simulink model "Collision_two_cars_cs"  (Simulink 8.7)
settings: Solver=ode5  SolverMode=SingleTasking  StartTime=0.0  StopTime=inf  FixedStep=1/20  RelTol=1e-3
PreLoadFcn:
  | check_NUTS_defined;
  | 
  | assignin('base',['model_closed_' bdroot],false);
InitFcn:
  | PreScanExperimentInitFcn(bdroot)
StopFcn:
  | PreScanExperimentStopFcn(bdroot)
undefined symbols (not defined in the file): spare_1, spare_10, spare_11, spare_12, spare_13, spare_14, spare_15, spare_16, spare_17, spare_18, spare_19, spare_2, spare_3, spare_4, spare_5, spare_6, spare_7, spare_8, spare_9
libraries: PreScanSimulinkLibrary x16, PreScanUsefulBlocks x6, simulink x1
(part 2 of 3)

== system Collision_two_cars_cs/STATE_Toyota_Yaris_1 ==
  State : Inport  SampleTime=TimeStep
  Acceleration : Subsystem  mask(ToSensorWorld){PortName=Acceleration_Toyota_Yaris_1, PortIndex=60, PortWidth=3, TimeStep=1/20}
      mask prompts: PortName "Port Name [-]"; PortIndex "Index [-]"; PortWidth "Port Dimensions [-]"; TimeStep "Upload Period [s]"
      mask help: Sends signal(s) from Simulink to the Sensor World
      mask Help:
      | Sends signal(s) from Simulink to the Sensor World.
      | 
      | - Port Name [-]: specifies the name of the output terminal of the Simulink block.
      | - Index [-]: specifies the start position in the output vector sent to the Sensor World
      | - Port dimensions [-]: specifies the width (number of scalars) of the output port
      | - Upload period [s]: specifies the upload period (in seconds) of the port.
      mask Display: port_label('input', 1, PortName)
  Demux : Demux  Outputs=5
  Position : Subsystem  mask(ToSensorWorld){PortName=Position_Toyota_Yaris_1, PortIndex=54, PortWidth=3, TimeStep=1/20}
      mask prompts: PortName "Port Name [-]"; PortIndex "Index [-]"; PortWidth "Port Dimensions [-]"; TimeStep "Upload Period [s]"
      mask help: Sends signal(s) from Simulink to the Sensor World
      mask Help:
      | Sends signal(s) from Simulink to the Sensor World.
      | 
      | - Port Name [-]: specifies the name of the output terminal of the Simulink block.
      | - Index [-]: specifies the start position in the output vector sent to the Sensor World
      | - Port dimensions [-]: specifies the width (number of scalars) of the output port
      | - Upload period [s]: specifies the upload period (in seconds) of the port.
      mask Display: port_label('input', 1, PortName)
  RPY : Subsystem  mask(ToSensorWorld){PortName=RPY_Toyota_Yaris_1, PortIndex=63, PortWidth=3, TimeStep=1/20}
      mask prompts: PortName "Port Name [-]"; PortIndex "Index [-]"; PortWidth "Port Dimensions [-]"; TimeStep "Upload Period [s]"
      mask help: Sends signal(s) from Simulink to the Sensor World
      mask Help:
      | Sends signal(s) from Simulink to the Sensor World.
      | 
      | - Port Name [-]: specifies the name of the output terminal of the Simulink block.
      | - Index [-]: specifies the start position in the output vector sent to the Sensor World
      | - Port dimensions [-]: specifies the width (number of scalars) of the output port
      | - Upload period [s]: specifies the upload period (in seconds) of the port.
      mask Display: port_label('input', 1, PortName)
  Velocity : Subsystem  mask(ToSensorWorld){PortName=Velocity_Toyota_Yaris_1, PortIndex=57, PortWidth=3, TimeStep=1/20}
      mask prompts: PortName "Port Name [-]"; PortIndex "Index [-]"; PortWidth "Port Dimensions [-]"; TimeStep "Upload Period [s]"
      mask help: Sends signal(s) from Simulink to the Sensor World
      mask Help:
      | Sends signal(s) from Simulink to the Sensor World.
      | 
      | - Port Name [-]: specifies the name of the output terminal of the Simulink block.
      | - Index [-]: specifies the start position in the output vector sent to the Sensor World
      | - Port dimensions [-]: specifies the width (number of scalars) of the output port
      | - Upload period [s]: specifies the upload period (in seconds) of the port.
      mask Display: port_label('input', 1, PortName)
  iniBODYAngles wrtVEH [rad] : Constant  Value=[Roll0 Pitch0 0]  SampleTime=TimeStep
  iniVEHAngles wrtGLOB [rad] : Constant  Value=[0 0 Yaw0]  SampleTime=TimeStep
  iniVEHposition wrtGLOB [m] : Constant  Value=[x0 y0 z0]  SampleTime=TimeStep
  state2FullState : PreScanSimulinkLibrary/state2FullState  SystemSampleTime=-1
  velRPY : Subsystem  mask(ToSensorWorld){PortName=velRPY_Toyota_Yaris_1, PortIndex=66, PortWidth=3, TimeStep=1/20}
      mask prompts: PortName "Port Name [-]"; PortIndex "Index [-]"; PortWidth "Port Dimensions [-]"; TimeStep "Upload Period [s]"
      mask help: Sends signal(s) from Simulink to the Sensor World
      mask Help:
      | Sends signal(s) from Simulink to the Sensor World.
      | 
      | - Port Name [-]: specifies the name of the output terminal of the Simulink block.
      | - Index [-]: specifies the start position in the output vector sent to the Sensor World
      | - Port dimensions [-]: specifies the width (number of scalars) of the output port
      | - Upload period [s]: specifies the upload period (in seconds) of the port.
      mask Display: port_label('input', 1, PortName)
  wires:
  Demux/5 -> velRPY/1(Y)
  Demux/4 -> RPY/1(Y)
  Demux/3 -> Acceleration/1(Y)
  Demux/2 -> Velocity/1(Y)
  Demux/1 -> Position/1(Y)
  State/1 -> state2FullState/1
  state2FullState/1 -> Demux/1
  iniVEHposition wrtGLOB [m]/1 -> state2FullState/2
  iniBODYAngles wrtVEH [rad]/1 -> state2FullState/3
  iniVEHAngles wrtGLOB [rad]/1 -> state2FullState/4

== system Collision_two_cars_cs/Scope Collision Detections ==
  In1 : Inport
  Collision Detections : Scope  NumInputPorts=5
  Demux2 : Demux  Outputs=5
  wires:
  Demux2/1 -> Collision Detections/1
  Demux2/2 -> Collision Detections/2
  Demux2/3 -> Collision Detections/3
  Demux2/4 -> Collision Detections/4
  Demux2/5 -> Collision Detections/5
  In1/1 -> Demux2/1

== system Collision_two_cars_cs/Scope Collision IDs ==
  In1 : Inport
  Collision IDs : Scope  NumInputPorts=5
  Demux2 : Demux  Outputs=5
  wires:
  In1/1 -> Demux2/1
  Demux2/5 -> Collision IDs/5
  Demux2/4 -> Collision IDs/4
  Demux2/3 -> Collision IDs/3
  Demux2/2 -> Collision IDs/2
  Demux2/1 -> Collision IDs/1

== system Collision_two_cars_cs/SetActuators ==
  Bus Creator : BusCreator  Inputs=1
  Data Store Read : DataStoreRead  DataStoreName=SimCoreActuators  SampleTime=TimeStep
  SendActuators : M-S-Function  FunctionName=SendActuatorsBlock  Parameters=TimeStep NrOfActuators
  dummy : Outport
  tag scope: SimCoreInfo=global
  wires:
  Bus Creator/1 -> [SimCoreInfo]  "SimCore"
  SendActuators/2 -> Bus Creator/1  "ComputationTime[s]"
  SendActuators/1 -> dummy/1
  Data Store Read/1 -> SendActuators/1

== system Collision_two_cars_cs/SimCoreInfo ==
  Bus Selector : BusSelector  OutputSignals=ComputationTime[s]
  Time : Scope
  wires:
  Bus Selector/1 -> Time/1  "<ComputationTime[s]>"
  [SimCoreInfo] -> Bus Selector/1

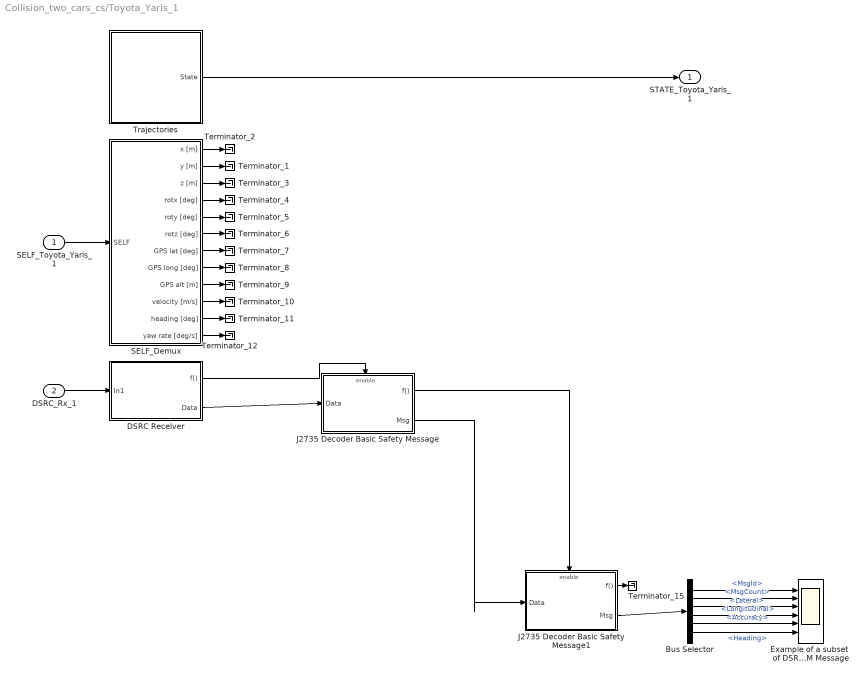
== system Collision_two_cars_cs/Toyota_Yaris_1 ==
  SELF_Toyota_Yaris_1 : Inport  Tag=SELFInport
  DSRC_Rx_1 : Inport  Tag=DSRC_RInport  Port=2
  Bus Selector : BusSelector  OutputSignals=MsgId,MsgCount,Lateral,Longitudinal,Accuracy,Heading
  DSRC Receiver : Subsystem  Tag=DSRC_Receiver
  Example of a subset  of DSRC Receiver BSM Message : Scope  NumInputPorts=6
  J2735 Decoder Basic Safety Message : Subsystem  Tag=J2735_Decoder_Basic_Safety_Message
  J2735 Decoder Basic Safety Message1 : Subsystem  Tag=J2735_Decoder_Basic_Safety_Message
  SELF_Demux : Subsystem  Tag=DemuxSELF  mask(PreScan Demux Block:){}
      settings: DeleteFcn=PreScanBlockDeleteFcn;
      mask Display:
      | port_label('output',1,'x [m]')
      | port_label('output',2,'y [m]')
      | port_label('output',3,'z [m]','texmode','on')
      | port_label('output',4,'Rotx [deg]','texmode','on')
      | port_label('output',5,'Roty [deg]','texmode','on')
      | port_label('output',6,'Rotz [deg]','texmode','on')
      | port_label('output',7,'GPS lat [deg]','texmode','on')
      | port_label('output',8,'GPS long [deg]','texmode','on')
      | port_label('output',9,'GPS alt [m]','texmode','on')
      | port_label('output',10,'Velocity [m/s]')
      | port_label('output',11,'Heading [deg]')
      | port_label('output',12,'Yaw rate [deg/s]')
  Terminator_{1..12,15} (13 alike) : Terminator
  Trajectories : Subsystem  Tag=Trajectories  mask(PreScan Source Block: Trajectories){}
      mask help:
      | The Trajectory block contains the trajectories defined in the PreScan Experiment Editor. The output of the trajectory block is the (vehicle) State.
      |
      | For more information, please click Help.
      settings: DeleteFcn=PreScanBlockDeleteFcn;
      mask Help: eval('openHelp(312)')
      mask Display: image(imread('Trajectory.png'));
  STATE_Toyota_Yaris_1 : Outport  Tag=StateOutport
  wires:
  J2735 Decoder Basic Safety Message/1(f()) -> J2735 Decoder Basic Safety Message1/Enable
  SELF_Demux/1(x [m]) -> Terminator_2/1
  SELF_Demux/2(y [m]) -> Terminator_1/1
  SELF_Demux/3(z [m]) -> Terminator_3/1
  SELF_Demux/4(rotx [deg]) -> Terminator_4/1
  SELF_Demux/5(roty [deg]) -> Terminator_5/1
  SELF_Demux/6(rotz [deg]) -> Terminator_6/1
  SELF_Demux/7(GPS lat [deg]) -> Terminator_7/1
  SELF_Demux/8(GPS long [deg]) -> Terminator_8/1
  SELF_Demux/9(GPS alt [m]) -> Terminator_9/1
  SELF_Demux/10(velocity [m/s]) -> Terminator_10/1
  SELF_Demux/11(heading [deg]) -> Terminator_11/1
  SELF_Demux/12(yaw rate [deg/s]) -> Terminator_12/1
  Bus Selector/1 -> Example of a subset  of DSRC Receiver BSM Message/1  "<MsgId>"
  Bus Selector/2 -> Example of a subset  of DSRC Receiver BSM Message/2  "<MsgCount>"
  Bus Selector/3 -> Example of a subset  of DSRC Receiver BSM Message/3  "<Lateral>"
  Bus Selector/4 -> Example of a subset  of DSRC Receiver BSM Message/4  "<Longitudinal>"
  Bus Selector/5 -> Example of a subset  of DSRC Receiver BSM Message/5  "<Accuracy>"
  J2735 Decoder Basic Safety Message1/2(Msg) -> Bus Selector/1
  J2735 Decoder Basic Safety Message1/1(f()) -> Terminator_15/1
  Bus Selector/6 -> Example of a subset  of DSRC Receiver BSM Message/6  "<Heading>"
  J2735 Decoder Basic Safety Message/2(Msg) -> J2735 Decoder Basic Safety Message1/1(Data)
  SELF_Toyota_Yaris_1/1 -> SELF_Demux/1(SELF)
  DSRC Receiver/1(f()) -> J2735 Decoder Basic Safety Message/Enable
  DSRC Receiver/2(Data) -> J2735 Decoder Basic Safety Message/1(Data)
  DSRC_Rx_1/1 -> DSRC Receiver/1(In1)
  Trajectories/1(State) -> STATE_Toyota_Yaris_1/1

== system Collision_two_cars_cs/Audi_A8_1/AIR_1_Demux ==
  AIR : Inport
  Activate_Switch : Subsystem
      mask Display: text(5,10,'')
  Bus Selector : BusSelector  OutputSignals=DATA.Range,DATA.Azimuth,DATA.Elevation,DATA.ID,DATA.Velocity,DATA.Heading
  Data Type Conversion : DataTypeConversion  OutDataTypeStr=double
  For Iterator : ForIterator  ResetStates=reset  IterationLimit=detectableObjects
  Selector : Selector  InputPortWidth=detectableObjects  IndexOptions=Index vector (port)  Indices=[1 3]  OutputSizes=1
  Signal2ArrayOfSignals1 : Subsystem  mask{VECTORLENGTH=detectableObjects}
      mask prompts: VECTORLENGTH "Length of vector"
  Signal2ArrayOfSignals2 : Subsystem  mask{VECTORLENGTH=detectableObjects}
      mask prompts: VECTORLENGTH "Length of vector"
  Signal2ArrayOfSignals3 : Subsystem  mask{VECTORLENGTH=detectableObjects}
      mask prompts: VECTORLENGTH "Length of vector"
  Signal2ArrayOfSignals4 : Subsystem  mask{VECTORLENGTH=detectableObjects}
      mask prompts: VECTORLENGTH "Length of vector"
  Signal2ArrayOfSignals5 : Subsystem  mask{VECTORLENGTH=detectableObjects}
      mask prompts: VECTORLENGTH "Length of vector"
  Signal2ArrayOfSignals6 : Subsystem  mask{VECTORLENGTH=detectableObjects}
      mask prompts: VECTORLENGTH "Length of vector"
  Range [m] : Outport
  Azimuth [deg] : Outport  Port=2
  Elevation [deg] : Outport  Port=3
  ID [-] : Outport  Port=4
  Velocity [m/s] : Outport  Port=5
  Heading [deg] : Outport  Port=6
  wires:
  Data Type Conversion/1 -> ID [-]/1
  Bus Selector/6 -> Signal2ArrayOfSignals6/2(Element)  "<Heading>"
  Signal2ArrayOfSignals6/1(ArrayofElements) -> Activate_Switch/2(Heading)
  Bus Selector/5 -> Signal2ArrayOfSignals5/2(Element)  "<Velocity>"
  Signal2ArrayOfSignals5/1(ArrayofElements) -> Velocity [m/s]/1
  Bus Selector/4 -> Signal2ArrayOfSignals4/2(Element)  "<ID>"
  Signal2ArrayOfSignals4/1(ArrayofElements) -> Data Type Conversion/1, Activate_Switch/1(BeamID)
  Bus Selector/3 -> Signal2ArrayOfSignals3/2(Element)  "<Elevation>"
  Signal2ArrayOfSignals3/1(ArrayofElements) -> Elevation [deg]/1
  Bus Selector/2 -> Signal2ArrayOfSignals1/2(Element)  "<Azimuth>"
  Signal2ArrayOfSignals1/1(ArrayofElements) -> Azimuth [deg]/1
  Signal2ArrayOfSignals2/1(ArrayofElements) -> Range [m]/1
  Bus Selector/1 -> Signal2ArrayOfSignals2/2(Element)  "<Range>"
  Selector/1 -> Bus Selector/1
  For Iterator/1 -> Signal2ArrayOfSignals6/1(LoopIndex), Signal2ArrayOfSignals5/1(LoopIndex), Signal2ArrayOfSignals4/1(LoopIndex), Signal2ArrayOfSignals3/1(LoopIndex), Signal2ArrayOfSignals1/1(LoopIndex), Signal2ArrayOfSignals2/1(LoopIndex), Selector/2
  AIR/1 -> Selector/1
  Activate_Switch/1(On/Off) -> Heading [deg]/1

== system Collision_two_cars_cs/Audi_A8_1/SELF_Demux ==
  SELF : Inport
  Demux1 : Demux  Outputs=3
  Demux2 : Demux  Outputs=3
  Demux3 : Demux  Outputs=[3 3 1 1]
  Demux4 : Demux  Outputs=3
  Gain : Gain  Gain=180/pi
  Gain1 : Gain  Gain=180/pi
  Selector : Selector  InputPortWidth=3  IndexOptions=Index vector (dialog)  Indices=[3]  OutputSizes=1
  compas converter : Subsystem
  xyz2GPS : PreScanUsefulBlocks/xyz2GPS  CoordinateCount=1  GPS_base=[48.534599 9.071365 0.000]
  x [m] : Outport
  y [m] : Outport  Port=2
  z [m] : Outport  Port=3
  rotx [deg] : Outport  Port=4
  roty [deg] : Outport  Port=5
  rotz [deg] : Outport  Port=6
  GPS lat [deg] : Outport  Port=7
  GPS long [deg] : Outport  Port=8
  GPS alt [m] : Outport  Port=9
  velocity [m/s] : Outport  Port=10
  heading [deg] : Outport  Port=11
  yaw rate [deg/s] : Outport  Port=12
  wires:
  Demux3/4 -> Gain1/1
  Gain1/1 -> yaw rate [deg/s]/1
  Demux3/3 -> velocity [m/s]/1
  compas converter/1(heading [deg]) -> heading [deg]/1
  xyz2GPS/1 -> Demux4/1
  Demux4/3 -> GPS alt [m]/1
  Demux4/2 -> GPS long [deg]/1
  Demux4/1 -> GPS lat [deg]/1
  Demux3/2 -> Gain/1, Selector/1
  Demux3/1 -> xyz2GPS/1, Demux1/1
  SELF/1 -> Demux3/1
  Demux2/3 -> rotz [deg]/1
  Demux2/2 -> roty [deg]/1
  Demux2/1 -> rotx [deg]/1
  Demux1/3 -> z [m]/1
  Demux1/2 -> y [m]/1
  Demux1/1 -> x [m]/1
  Gain/1 -> Demux2/1
  Selector/1 -> compas converter/1(rotz [rad])

== system Collision_two_cars_cs/Audi_A8_1/Trajectories ==
  Traj2State1 : Subsystem  Tag=Traj2State  mask(PreScan Demux Block:){}
      settings: DeleteFcn=PreScanBlockDeleteFcn;
  Trajectory_1 : Subsystem  Tag=Trajectory  mask(PreScan Source Block: Trajectory){FileName='Trajectory_1_Synced.mat', TimeStep=1/20}
      mask prompts: TimeStep "Time Step [s]"
      mask help:
      | The Trajectory block contains the trajectories defined in the PreScan Experiment Editor. The output of the trajectory block is the (vehicle) State.
      |
      | For more information, please click Help.
      mask init:
      | [direc,name]=fileparts(get_param(bdroot, 'FileName'));
      | load([direc,'/Trajectories/',FileName])
      | trajectory=trajectory';
      | 
      | traj.time=trajectory(:,1);%[];
      | traj.signals.values=trajectory(:,2:19);
      | traj.dimensions=18;
      | traj.label='';
      | 
      | SampleTime=traj.time(2)-traj.time(1);
      settings: DeleteFcn=PreScanBlockDeleteFcn;
      mask Help: eval('openHelp(312)')
      mask Display: fprintf(FileName)
  Trajectory_1_Offset : Constant  Tag=TrajectoryOffset  Value="[0  0  0  0  0  0]"
  State : Outport  Tag=TrajOutport
  wires:
  Trajectory_1/1(trajectory) -> Traj2State1/1(Traj Org)
  Trajectory_1_Offset/1 -> Traj2State1/2(Offset)
  Traj2State1/1(state) -> State/1

== system Collision_two_cars_cs/BMW_X5_1/DSRC Transmitter ==
  Data : Inport
  Enable : EnablePort  PropagateVarSize=During execution
  DSRC_T_BusAssignment : BusAssignment  Tag=BusDSRCT  AssignedSignals=spare_1,spare_2,spare_3,spare_4,spare_5,spare_6,spare_7,spare_8,spare_9,spare_10,spare_11,spare_12,spare_13,spare_14,spare_15,spare_16,spare_17,spare_18,spare_19
  DSRC_T_Mux : Subsystem  Tag=MuxDSRCT  mask(PreScan Mux Block:){}
      settings: DeleteFcn=PreScanBlockDeleteFcn;
      mask Display:
      | port_label('input', 1, 'Warning signal ID')
      | port_label('input', 2, 'Maneuvre ID')
      | port_label('input', 3, 'Vehicle Type')
      | port_label('input', 4, 'Braking Capacity')
      | port_label('input', 5, 'Vehicle Size')
      | port_label('input', 6, 'spare')
  Demux : Demux  Outputs=19
  Ground_{4..8} (5 alike) : Ground
  DSRC_T : Outport  Tag=AntennaTOutport
  wires:
  Demux/19 -> DSRC_T_BusAssignment/20  "Vehicle Height"
  Demux/18 -> DSRC_T_BusAssignment/19  "Vehicle Width"
  Demux/17 -> DSRC_T_BusAssignment/18  "Brakes"
  Demux/16 -> DSRC_T_BusAssignment/17  "Yaw rate"
  Demux/15 -> DSRC_T_BusAssignment/16  "Veritical Acc"
  Demux/14 -> DSRC_T_BusAssignment/15  "Lateral Acc"
  Demux/13 -> DSRC_T_BusAssignment/14  "Longitudinal Acc"
  Demux/12 -> DSRC_T_BusAssignment/13  "Angle"
  Demux/11 -> DSRC_T_BusAssignment/12  "Heading"
  Demux/10 -> DSRC_T_BusAssignment/11  "Speed"
  Demux/9 -> DSRC_T_BusAssignment/10  "Transmission State"
  Demux/8 -> DSRC_T_BusAssignment/9  "Accuracy"
  Demux/7 -> DSRC_T_BusAssignment/8  "Elevation"
  Demux/6 -> DSRC_T_BusAssignment/7  "Longitudinal"
  Demux/5 -> DSRC_T_BusAssignment/6  "Lateral"
  Ground_8/1 -> DSRC_T_Mux/5(vehicle_size)  "l50"
  Ground_7/1 -> DSRC_T_Mux/4(brakingcapacity)  "l49"
  Ground_6/1 -> DSRC_T_Mux/3(vehicle_type)  "l48"
  Ground_5/1 -> DSRC_T_Mux/2(maneuvre_id)  "l47"
  Ground_4/1 -> DSRC_T_Mux/1(warning_signal_id)  "l46"
  DSRC_T_Mux/1(Out1) -> DSRC_T/1  "l60"
  DSRC_T_BusAssignment/1 -> DSRC_T_Mux/6(spare)  "l58"
  Demux/4 -> DSRC_T_BusAssignment/5  "SecMark"
  Demux/3 -> DSRC_T_BusAssignment/4  "TempId"
  Demux/2 -> DSRC_T_BusAssignment/3  "MsgCount"
  Demux/1 -> DSRC_T_BusAssignment/2  "MsgId"
  Data/1 -> Demux/1
  DSRC_T_Mux/2(Out2) -> DSRC_T_BusAssignment/1  "L29"

== system Collision_two_cars_cs/BMW_X5_1/J2735 Encoder Basic Safety Message ==
  Msg : Inport
  Enable : EnablePort  PropagateVarSize=During execution
  Constant : Constant
  Demux : Demux  Outputs=19
  Embedded MATLAB Function : MATLAB Function  TreatAsAtomicUnit=on
  f() : Outport  InitialOutput=[1]
  Data : Outport  Port=2
  wires:
  Embedded MATLAB Function/1(y) -> Data/1
  Demux/19 -> Embedded MATLAB Function/19(u19)
  Demux/18 -> Embedded MATLAB Function/18(u18)
  Demux/17 -> Embedded MATLAB Function/17(u17)
  Demux/16 -> Embedded MATLAB Function/16(u16)
  Demux/15 -> Embedded MATLAB Function/15(u15)
  Demux/14 -> Embedded MATLAB Function/14(u14)
  Demux/13 -> Embedded MATLAB Function/13(u13)
  Demux/12 -> Embedded MATLAB Function/12(u12)
  Demux/11 -> Embedded MATLAB Function/11(u11)
  Demux/10 -> Embedded MATLAB Function/10(u10)
  Demux/9 -> Embedded MATLAB Function/9(u9)
  Demux/8 -> Embedded MATLAB Function/8(u8)
  Demux/7 -> Embedded MATLAB Function/7(u7)
  Demux/6 -> Embedded MATLAB Function/6(u6)
  Demux/5 -> Embedded MATLAB Function/5(u5)
  Demux/4 -> Embedded MATLAB Function/4(u4)
  Demux/3 -> Embedded MATLAB Function/3(u3)
  Demux/2 -> Embedded MATLAB Function/2(u2)
  Demux/1 -> Embedded MATLAB Function/1(u1)
  Constant/1 -> f()/1  "Enabled"
  Msg/1 -> Demux/1

== system Collision_two_cars_cs/BMW_X5_1/SELF_Demux ==
  SELF : Inport
  Demux1 : Demux  Outputs=3
  Demux2 : Demux  Outputs=3
  Demux3 : Demux  Outputs=[3 3 1 1]
  Demux4 : Demux  Outputs=3
  Gain : Gain  Gain=180/pi
  Gain1 : Gain  Gain=180/pi
  Selector : Selector  InputPortWidth=3  IndexOptions=Index vector (dialog)  Indices=[3]  OutputSizes=1
  compas converter : Subsystem
  xyz2GPS : PreScanUsefulBlocks/xyz2GPS  CoordinateCount=1  GPS_base=[48.534599 9.071365 0.000]
  x [m] : Outport
  y [m] : Outport  Port=2
  z [m] : Outport  Port=3
  rotx [deg] : Outport  Port=4
  roty [deg] : Outport  Port=5
  rotz [deg] : Outport  Port=6
  GPS lat [deg] : Outport  Port=7
  GPS long [deg] : Outport  Port=8
  GPS alt [m] : Outport  Port=9
  velocity [m/s] : Outport  Port=10
  heading [deg] : Outport  Port=11
  yaw rate [deg/s] : Outport  Port=12
  wires:
  Demux3/4 -> Gain1/1
  Gain1/1 -> yaw rate [deg/s]/1
  Demux3/3 -> velocity [m/s]/1
  compas converter/1(heading [deg]) -> heading [deg]/1
  xyz2GPS/1 -> Demux4/1
  Demux4/3 -> GPS alt [m]/1
  Demux4/2 -> GPS long [deg]/1
  Demux4/1 -> GPS lat [deg]/1
  Demux3/2 -> Gain/1, Selector/1
  Demux3/1 -> xyz2GPS/1, Demux1/1
  SELF/1 -> Demux3/1
  Demux2/3 -> rotz [deg]/1
  Demux2/2 -> roty [deg]/1
  Demux2/1 -> rotx [deg]/1
  Demux1/3 -> z [m]/1
  Demux1/2 -> y [m]/1
  Demux1/1 -> x [m]/1
  Gain/1 -> Demux2/1
  Selector/1 -> compas converter/1(rotz [rad])

== system Collision_two_cars_cs/BMW_X5_1/Trajectories ==
  Traj2State1 : Subsystem  Tag=Traj2State  mask(PreScan Demux Block:){}
      settings: DeleteFcn=PreScanBlockDeleteFcn;
  Trajectory_2 : Subsystem  Tag=Trajectory  mask(PreScan Source Block: Trajectory){FileName='Trajectory_2_Synced.mat', TimeStep=1/20}
      mask prompts: TimeStep "Time Step [s]"
      mask help:
      | The Trajectory block contains the trajectories defined in the PreScan Experiment Editor. The output of the trajectory block is the (vehicle) State.
      |
      | For more information, please click Help.
      mask init: same as Collision_two_cars_cs/Audi_A8_1/Trajectories/Trajectory_1
      settings: DeleteFcn=PreScanBlockDeleteFcn;
      mask Help: eval('openHelp(312)')
      mask Display: fprintf(FileName)
  Trajectory_2_Offset : Constant  Tag=TrajectoryOffset  Value="[0  0  0  0  0  0]"
  State : Outport  Tag=TrajOutport
  wires:
  Trajectory_2/1(trajectory) -> Traj2State1/1(Traj Org)
  Trajectory_2_Offset/1 -> Traj2State1/2(Offset)
  Traj2State1/1(state) -> State/1

== system Collision_two_cars_cs/Citroen_C3_1/SELF_Demux ==
  SELF : Inport
  Demux1 : Demux  Outputs=3
  Demux2 : Demux  Outputs=3
  Demux3 : Demux  Outputs=[3 3 1 1]
  Demux4 : Demux  Outputs=3
  Gain : Gain  Gain=180/pi
  Gain1 : Gain  Gain=180/pi
  Selector : Selector  InputPortWidth=3  IndexOptions=Index vector (dialog)  Indices=[3]  OutputSizes=1
  compas converter : Subsystem
  xyz2GPS : PreScanUsefulBlocks/xyz2GPS  CoordinateCount=1  GPS_base=[48.534599 9.071365 0.000]
  x [m] : Outport
  y [m] : Outport  Port=2
  z [m] : Outport  Port=3
  rotx [deg] : Outport  Port=4
  roty [deg] : Outport  Port=5
  rotz [deg] : Outport  Port=6
  GPS lat [deg] : Outport  Port=7
  GPS long [deg] : Outport  Port=8
  GPS alt [m] : Outport  Port=9
  velocity [m/s] : Outport  Port=10
  heading [deg] : Outport  Port=11
  yaw rate [deg/s] : Outport  Port=12
  wires:
  Demux3/4 -> Gain1/1
  Gain1/1 -> yaw rate [deg/s]/1
  Demux3/3 -> velocity [m/s]/1
  compas converter/1(heading [deg]) -> heading [deg]/1
  xyz2GPS/1 -> Demux4/1
  Demux4/3 -> GPS alt [m]/1
  Demux4/2 -> GPS long [deg]/1
  Demux4/1 -> GPS lat [deg]/1
  Demux3/2 -> Gain/1, Selector/1
  Demux3/1 -> xyz2GPS/1, Demux1/1
  SELF/1 -> Demux3/1
  Demux2/3 -> rotz [deg]/1
  Demux2/2 -> roty [deg]/1
  Demux2/1 -> rotx [deg]/1
  Demux1/3 -> z [m]/1
  Demux1/2 -> y [m]/1
  Demux1/1 -> x [m]/1
  Gain/1 -> Demux2/1
  Selector/1 -> compas converter/1(rotz [rad])

== system Collision_two_cars_cs/Citroen_C3_1/TIS_1_Standard_Demux ==
  Radar : Inport
  Bus Creator : BusCreator  Inputs=6
  Bus Selector : BusSelector  OutputSignals=ActiveBeamID[-],Range[m],Theta[deg],Phi[deg],TargetID[-],TargetTypeID[-]
  ScannerSensorLegacyBusConversion : PreScanUsefulBlocks/ScannerSensorLegacyBusConversion  MAXMESSAGES=MAXMESSAGES
  Out1 : Outport
  Out2 : Outport  Port=2
  Out3 : Outport  Port=3
  Out4 : Outport  Port=4
  Out5 : Outport  Port=5
  Out6 : Outport  Port=6
  wires:
  Bus Selector/2 -> Bus Creator/2, Out2/1  "<Range[m]>"
  Bus Selector/1 -> Bus Creator/1, Out1/1  "<ActiveBeamID[-]>"
  ScannerSensorLegacyBusConversion/1 -> Bus Selector/1
  Radar/1 -> ScannerSensorLegacyBusConversion/1
  Bus Selector/6 -> Bus Creator/6  "<TargetTypeID[-]>"
  Bus Creator/1 -> Out6/1
  Bus Selector/5 -> Bus Creator/5, Out5/1  "<TargetID[-]>"
  Bus Selector/4 -> Out4/1, Bus Creator/4  "<Phi[deg]>"
  Bus Selector/3 -> Out3/1, Bus Creator/3  "<Theta[deg]>"

== system Collision_two_cars_cs/Citroen_C3_1/Trajectories ==
  Traj2State1 : Subsystem  Tag=Traj2State  mask(PreScan Demux Block:){}
      settings: DeleteFcn=PreScanBlockDeleteFcn;
  Trajectory_4 : Subsystem  Tag=Trajectory  mask(PreScan Source Block: Trajectory){FileName='Trajectory_4_Synced.mat', TimeStep=1/20}
      mask prompts: TimeStep "Time Step [s]"
      mask help:
      | The Trajectory block contains the trajectories defined in the PreScan Experiment Editor. The output of the trajectory block is the (vehicle) State.
      |
      | For more information, please click Help.
      mask init: same as Collision_two_cars_cs/Audi_A8_1/Trajectories/Trajectory_1
      settings: DeleteFcn=PreScanBlockDeleteFcn;
      mask Help: eval('openHelp(312)')
      mask Display: fprintf(FileName)
  Trajectory_4_Offset : Constant  Tag=TrajectoryOffset  Value="[0  0  0  0  0  0]"
  State : Outport  Tag=TrajOutport
  wires:
  Trajectory_4/1(trajectory) -> Traj2State1/1(Traj Org)
  Trajectory_4_Offset/1 -> Traj2State1/2(Offset)
  Traj2State1/1(state) -> State/1

== system Collision_two_cars_cs/CollisionDetection/retrieve CollisionDetection signal ==
  In : Inport
  Constant1 : Constant  Value=0
  Relational Operator : RelationalOperator  Operator=>  OutDataTypeStr=boolean
  Selector : Selector  InputPortWidth=10  IndexOptions=Index vector (dialog)  Indices=[1 3 5 7 9]  OutputSizes=1
  Out : Outport
  wires:
  Relational Operator/1 -> Out/1
  In/1 -> Selector/1
  Selector/1 -> Relational Operator/1
  Constant1/1 -> Relational Operator/2

== system Collision_two_cars_cs/STATE_Audi_A8_1/Acceleration ==
  Y : Inport
  Assignment : Assignment  IndexMode=Zero-based  SampleTime=TimeStep  IndexOptions=Starting index (dialog)  Indices=PortIndex  OutputSizes=[1 1]
  Data Store Read : DataStoreRead  DataStoreName=SimCoreActuators  SampleTime=TimeStep
  Data Store Write : DataStoreWrite  DataStoreName=SimCoreActuators
  wires:
  Assignment/1 -> Data Store Write/1
  Data Store Read/1 -> Assignment/1
  Y/1 -> Assignment/2

== system Collision_two_cars_cs/STATE_Audi_A8_1/Position ==
  Y : Inport
  Assignment : Assignment  IndexMode=Zero-based  SampleTime=TimeStep  IndexOptions=Starting index (dialog)  Indices=PortIndex  OutputSizes=[1 1]
  Data Store Read : DataStoreRead  DataStoreName=SimCoreActuators  SampleTime=TimeStep
  Data Store Write : DataStoreWrite  DataStoreName=SimCoreActuators
  wires:
  Y/1 -> Assignment/2
  Data Store Read/1 -> Assignment/1
  Assignment/1 -> Data Store Write/1

== system Collision_two_cars_cs/STATE_Audi_A8_1/RPY ==
  Y : Inport
  Assignment : Assignment  IndexMode=Zero-based  SampleTime=TimeStep  IndexOptions=Starting index (dialog)  Indices=PortIndex  OutputSizes=[1 1]
  Data Store Read : DataStoreRead  DataStoreName=SimCoreActuators  SampleTime=TimeStep
  Data Store Write : DataStoreWrite  DataStoreName=SimCoreActuators
  wires:
  Assignment/1 -> Data Store Write/1
  Data Store Read/1 -> Assignment/1
  Y/1 -> Assignment/2

== system Collision_two_cars_cs/STATE_Audi_A8_1/Velocity ==
  Y : Inport
  Assignment : Assignment  IndexMode=Zero-based  SampleTime=TimeStep  IndexOptions=Starting index (dialog)  Indices=PortIndex  OutputSizes=[1 1]
  Data Store Read : DataStoreRead  DataStoreName=SimCoreActuators  SampleTime=TimeStep
  Data Store Write : DataStoreWrite  DataStoreName=SimCoreActuators
  wires:
  Assignment/1 -> Data Store Write/1
  Data Store Read/1 -> Assignment/1
  Y/1 -> Assignment/2

== system Collision_two_cars_cs/STATE_Audi_A8_1/velRPY ==
  Y : Inport
  Assignment : Assignment  IndexMode=Zero-based  SampleTime=TimeStep  IndexOptions=Starting index (dialog)  Indices=PortIndex  OutputSizes=[1 1]
  Data Store Read : DataStoreRead  DataStoreName=SimCoreActuators  SampleTime=TimeStep
  Data Store Write : DataStoreWrite  DataStoreName=SimCoreActuators
  wires:
  Assignment/1 -> Data Store Write/1
  Data Store Read/1 -> Assignment/1
  Y/1 -> Assignment/2

== system Collision_two_cars_cs/STATE_BMW_X5_1/Acceleration ==
  Y : Inport
  Assignment : Assignment  IndexMode=Zero-based  SampleTime=TimeStep  IndexOptions=Starting index (dialog)  Indices=PortIndex  OutputSizes=[1 1]
  Data Store Read : DataStoreRead  DataStoreName=SimCoreActuators  SampleTime=TimeStep
  Data Store Write : DataStoreWrite  DataStoreName=SimCoreActuators
  wires:
  Assignment/1 -> Data Store Write/1
  Data Store Read/1 -> Assignment/1
  Y/1 -> Assignment/2

== system Collision_two_cars_cs/STATE_BMW_X5_1/Position ==
  Y : Inport
  Assignment : Assignment  IndexMode=Zero-based  SampleTime=TimeStep  IndexOptions=Starting index (dialog)  Indices=PortIndex  OutputSizes=[1 1]
  Data Store Read : DataStoreRead  DataStoreName=SimCoreActuators  SampleTime=TimeStep
  Data Store Write : DataStoreWrite  DataStoreName=SimCoreActuators
  wires:
  Y/1 -> Assignment/2
  Data Store Read/1 -> Assignment/1
  Assignment/1 -> Data Store Write/1

== system Collision_two_cars_cs/STATE_BMW_X5_1/RPY ==
  Y : Inport
  Assignment : Assignment  IndexMode=Zero-based  SampleTime=TimeStep  IndexOptions=Starting index (dialog)  Indices=PortIndex  OutputSizes=[1 1]
  Data Store Read : DataStoreRead  DataStoreName=SimCoreActuators  SampleTime=TimeStep
  Data Store Write : DataStoreWrite  DataStoreName=SimCoreActuators
  wires:
  Assignment/1 -> Data Store Write/1
  Data Store Read/1 -> Assignment/1
  Y/1 -> Assignment/2

== system Collision_two_cars_cs/STATE_BMW_X5_1/Velocity ==
  Y : Inport
  Assignment : Assignment  IndexMode=Zero-based  SampleTime=TimeStep  IndexOptions=Starting index (dialog)  Indices=PortIndex  OutputSizes=[1 1]
  Data Store Read : DataStoreRead  DataStoreName=SimCoreActuators  SampleTime=TimeStep
  Data Store Write : DataStoreWrite  DataStoreName=SimCoreActuators
  wires:
  Assignment/1 -> Data Store Write/1
  Data Store Read/1 -> Assignment/1
  Y/1 -> Assignment/2

== system Collision_two_cars_cs/STATE_BMW_X5_1/velRPY ==
  Y : Inport
  Assignment : Assignment  IndexMode=Zero-based  SampleTime=TimeStep  IndexOptions=Starting index (dialog)  Indices=PortIndex  OutputSizes=[1 1]
  Data Store Read : DataStoreRead  DataStoreName=SimCoreActuators  SampleTime=TimeStep
  Data Store Write : DataStoreWrite  DataStoreName=SimCoreActuators
  wires:
  Assignment/1 -> Data Store Write/1
  Data Store Read/1 -> Assignment/1
  Y/1 -> Assignment/2

== system Collision_two_cars_cs/STATE_Citroen_C3_1/Acceleration ==
  Y : Inport
  Assignment : Assignment  IndexMode=Zero-based  SampleTime=TimeStep  IndexOptions=Starting index (dialog)  Indices=PortIndex  OutputSizes=[1 1]
  Data Store Read : DataStoreRead  DataStoreName=SimCoreActuators  SampleTime=TimeStep
  Data Store Write : DataStoreWrite  DataStoreName=SimCoreActuators
  wires:
  Assignment/1 -> Data Store Write/1
  Data Store Read/1 -> Assignment/1
  Y/1 -> Assignment/2

== system Collision_two_cars_cs/STATE_Citroen_C3_1/Position ==
  Y : Inport
  Assignment : Assignment  IndexMode=Zero-based  SampleTime=TimeStep  IndexOptions=Starting index (dialog)  Indices=PortIndex  OutputSizes=[1 1]
  Data Store Read : DataStoreRead  DataStoreName=SimCoreActuators  SampleTime=TimeStep
  Data Store Write : DataStoreWrite  DataStoreName=SimCoreActuators
  wires:
  Y/1 -> Assignment/2
  Data Store Read/1 -> Assignment/1
  Assignment/1 -> Data Store Write/1

== system Collision_two_cars_cs/STATE_Citroen_C3_1/RPY ==
  Y : Inport
  Assignment : Assignment  IndexMode=Zero-based  SampleTime=TimeStep  IndexOptions=Starting index (dialog)  Indices=PortIndex  OutputSizes=[1 1]
  Data Store Read : DataStoreRead  DataStoreName=SimCoreActuators  SampleTime=TimeStep
  Data Store Write : DataStoreWrite  DataStoreName=SimCoreActuators
  wires:
  Assignment/1 -> Data Store Write/1
  Data Store Read/1 -> Assignment/1
  Y/1 -> Assignment/2

== system Collision_two_cars_cs/STATE_Citroen_C3_1/Velocity ==
  Y : Inport
  Assignment : Assignment  IndexMode=Zero-based  SampleTime=TimeStep  IndexOptions=Starting index (dialog)  Indices=PortIndex  OutputSizes=[1 1]
  Data Store Read : DataStoreRead  DataStoreName=SimCoreActuators  SampleTime=TimeStep
  Data Store Write : DataStoreWrite  DataStoreName=SimCoreActuators
  wires:
  Assignment/1 -> Data Store Write/1
  Data Store Read/1 -> Assignment/1
  Y/1 -> Assignment/2

== system Collision_two_cars_cs/STATE_Citroen_C3_1/velRPY ==
  Y : Inport
  Assignment : Assignment  IndexMode=Zero-based  SampleTime=TimeStep  IndexOptions=Starting index (dialog)  Indices=PortIndex  OutputSizes=[1 1]
  Data Store Read : DataStoreRead  DataStoreName=SimCoreActuators  SampleTime=TimeStep
  Data Store Write : DataStoreWrite  DataStoreName=SimCoreActuators
  wires:
  Assignment/1 -> Data Store Write/1
  Data Store Read/1 -> Assignment/1
  Y/1 -> Assignment/2

== system Collision_two_cars_cs/STATE_Toyota_Yaris_1/Acceleration ==
  Y : Inport
  Assignment : Assignment  IndexMode=Zero-based  SampleTime=TimeStep  IndexOptions=Starting index (dialog)  Indices=PortIndex  OutputSizes=[1 1]
  Data Store Read : DataStoreRead  DataStoreName=SimCoreActuators  SampleTime=TimeStep
  Data Store Write : DataStoreWrite  DataStoreName=SimCoreActuators
  wires:
  Assignment/1 -> Data Store Write/1
  Data Store Read/1 -> Assignment/1
  Y/1 -> Assignment/2

== system Collision_two_cars_cs/STATE_Toyota_Yaris_1/Position ==
  Y : Inport
  Assignment : Assignment  IndexMode=Zero-based  SampleTime=TimeStep  IndexOptions=Starting index (dialog)  Indices=PortIndex  OutputSizes=[1 1]
  Data Store Read : DataStoreRead  DataStoreName=SimCoreActuators  SampleTime=TimeStep
  Data Store Write : DataStoreWrite  DataStoreName=SimCoreActuators
  wires:
  Y/1 -> Assignment/2
  Data Store Read/1 -> Assignment/1
  Assignment/1 -> Data Store Write/1

== system Collision_two_cars_cs/STATE_Toyota_Yaris_1/RPY ==
  Y : Inport
  Assignment : Assignment  IndexMode=Zero-based  SampleTime=TimeStep  IndexOptions=Starting index (dialog)  Indices=PortIndex  OutputSizes=[1 1]
  Data Store Read : DataStoreRead  DataStoreName=SimCoreActuators  SampleTime=TimeStep
  Data Store Write : DataStoreWrite  DataStoreName=SimCoreActuators
  wires:
  Assignment/1 -> Data Store Write/1
  Data Store Read/1 -> Assignment/1
  Y/1 -> Assignment/2

== system Collision_two_cars_cs/STATE_Toyota_Yaris_1/Velocity ==
  Y : Inport
  Assignment : Assignment  IndexMode=Zero-based  SampleTime=TimeStep  IndexOptions=Starting index (dialog)  Indices=PortIndex  OutputSizes=[1 1]
  Data Store Read : DataStoreRead  DataStoreName=SimCoreActuators  SampleTime=TimeStep
  Data Store Write : DataStoreWrite  DataStoreName=SimCoreActuators
  wires:
  Assignment/1 -> Data Store Write/1
  Data Store Read/1 -> Assignment/1
  Y/1 -> Assignment/2

== system Collision_two_cars_cs/STATE_Toyota_Yaris_1/velRPY ==
  Y : Inport
  Assignment : Assignment  IndexMode=Zero-based  SampleTime=TimeStep  IndexOptions=Starting index (dialog)  Indices=PortIndex  OutputSizes=[1 1]
  Data Store Read : DataStoreRead  DataStoreName=SimCoreActuators  SampleTime=TimeStep
  Data Store Write : DataStoreWrite  DataStoreName=SimCoreActuators
  wires:
  Assignment/1 -> Data Store Write/1
  Data Store Read/1 -> Assignment/1
  Y/1 -> Assignment/2

== system Collision_two_cars_cs/Toyota_Yaris_1/DSRC Receiver ==
  In1 : Inport
  Always Enabled : Constant
  Bus Selector : BusSelector  OutputSignals=spare_1,spare_2,spare_3,spare_4,spare_5,spare_6,spare_7,spare_8,spare_9,spare_10,spare_11,spare_12,spare_13,spare_14,spare_15,spare_16,spare_17,spare_18,spare_19  OutputAsBus=on
  Bus to Vector : BusToVector
  DSRC_Rx_Demux : Subsystem  Tag=DemuxDSRCR  mask(PreScan Demux Block:){}
      settings: DeleteFcn=PreScanBlockDeleteFcn;
      mask Display:
      | port_label('output', 1, 'Vehicle_ID')
      | port_label('output', 2, 'GPS Pos Lat [deg]')
      | port_label('output', 3, 'GPS Pos Long [deg]')
      | port_label('output', 4, 'GPS Pos Alt [m]')
      | port_label('output', 5, 'Velocity [m/s]')
      | port_label('output', 6, 'Acceleration [m/s2]')
      | port_label('output', 7, 'Heading [deg]')
      | port_label('output', 8, 'Warning signal ID')
      | port_label('output', 9, 'Maneuvre ID')
      | port_label('output', 10, 'Vehicle Type')
      | port_label('output', 11, 'Braking Capacity')
      | port_label('output', 12, 'Vehicle Size')
      | port_label('output', 13, 'Spare')
  Terminator_{2..13} (12 alike) : Terminator
  f() : Outport
  Data : Outport  Port=2
  wires:
  Bus to Vector/1 -> Data/1
  Bus Selector/1 -> Bus to Vector/1
  DSRC_Rx_Demux/13(spare) -> Bus Selector/1  "L7"
  Always Enabled/1 -> f()/1  "Enable"
  In1/1 -> DSRC_Rx_Demux/1(AntennaR)
  DSRC_Rx_Demux/12(vehicle_size) -> Terminator_13/1
  DSRC_Rx_Demux/11(brakingcapacity) -> Terminator_12/1
  DSRC_Rx_Demux/10(vehicle_type) -> Terminator_11/1
  DSRC_Rx_Demux/9(maneuvre_id) -> Terminator_10/1
  DSRC_Rx_Demux/8(warning_signal_id) -> Terminator_9/1
  DSRC_Rx_Demux/7(Heading [deg]) -> Terminator_8/1
  DSRC_Rx_Demux/6(Acceleration_[m/s2]) -> Terminator_7/1
  DSRC_Rx_Demux/5(Velocity_[m/s]) -> Terminator_6/1
  DSRC_Rx_Demux/4(GPS_pos_alt_[m]) -> Terminator_5/1
  DSRC_Rx_Demux/3(GPS_pos_long_[deg]) -> Terminator_4/1
  DSRC_Rx_Demux/2(GPS_pos_lat_[deg]) -> Terminator_3/1
  DSRC_Rx_Demux/1(Vehicle_ID) -> Terminator_2/1

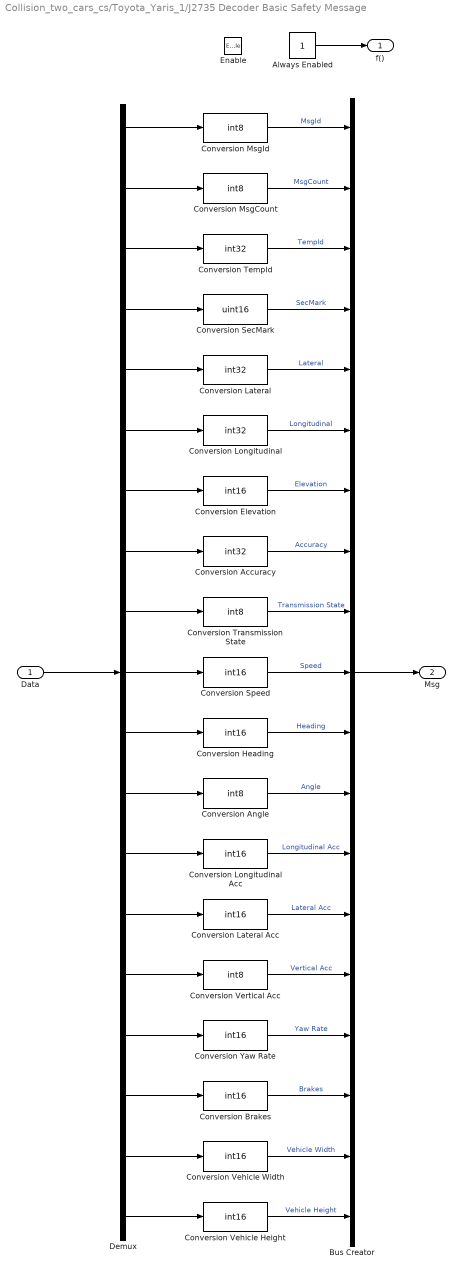
== system Collision_two_cars_cs/Toyota_Yaris_1/J2735 Decoder Basic Safety Message ==
  Data : Inport
  Enable : EnablePort  PropagateVarSize=During execution
  Always Enabled : Constant
  Bus Creator : BusCreator  Inputs=19
  Conversion Accuracy : DataTypeConversion  OutDataTypeStr=int32
  Conversion Angle : DataTypeConversion  OutDataTypeStr=int8
  Conversion Brakes : DataTypeConversion  OutDataTypeStr=int16
  Conversion Elevation : DataTypeConversion  OutDataTypeStr=int16
  Conversion Heading : DataTypeConversion  OutDataTypeStr=int16
  Conversion Lateral : DataTypeConversion  OutDataTypeStr=int32
  Conversion Lateral Acc : DataTypeConversion  OutDataTypeStr=int16
  Conversion Longitudinal : DataTypeConversion  OutDataTypeStr=int32
  Conversion Longitudinal Acc : DataTypeConversion  OutDataTypeStr=int16
  Conversion MsgCount : DataTypeConversion  OutDataTypeStr=int8
  Conversion MsgId : DataTypeConversion  OutDataTypeStr=int8
  Conversion SecMark : DataTypeConversion  OutDataTypeStr=uint16
  Conversion Speed : DataTypeConversion  OutDataTypeStr=int16
  Conversion TempId : DataTypeConversion  OutDataTypeStr=int32
  Conversion Transmission State : DataTypeConversion  OutDataTypeStr=int8
  Conversion Vehicle Height : DataTypeConversion  OutDataTypeStr=int16
  Conversion Vehicle Width : DataTypeConversion  OutDataTypeStr=int16
  Conversion Vertical Acc : DataTypeConversion  OutDataTypeStr=int8
  Conversion Yaw Rate : DataTypeConversion  OutDataTypeStr=int16
  Demux : Demux  Outputs=19
  f() : Outport  InitialOutput=[1]
  Msg : Outport  Port=2
  wires:
  Conversion Vehicle Height/1 -> Bus Creator/19  "Vehicle Height"
  Demux/19 -> Conversion Vehicle Height/1
  Conversion Vehicle Width/1 -> Bus Creator/18  "Vehicle Width"
  Conversion Brakes/1 -> Bus Creator/17  "Brakes"
  Demux/18 -> Conversion Vehicle Width/1
  Demux/17 -> Conversion Brakes/1
  Conversion Yaw Rate/1 -> Bus Creator/16  "Yaw Rate"
  Conversion Vertical Acc/1 -> Bus Creator/15  "Vertical Acc"
  Demux/16 -> Conversion Yaw Rate/1
  Demux/15 -> Conversion Vertical Acc/1
  Conversion Lateral Acc/1 -> Bus Creator/14  "Lateral Acc"
  Conversion Longitudinal Acc/1 -> Bus Creator/13  "Longitudinal Acc"
  Demux/14 -> Conversion Lateral Acc/1
  Demux/13 -> Conversion Longitudinal Acc/1
  Conversion Angle/1 -> Bus Creator/12  "Angle"
  Conversion Heading/1 -> Bus Creator/11  "Heading"
  Demux/12 -> Conversion Angle/1
  Demux/11 -> Conversion Heading/1
  Conversion Speed/1 -> Bus Creator/10  "Speed"
  Conversion Transmission State/1 -> Bus Creator/9  "Transmission State"
  Demux/10 -> Conversion Speed/1
  Demux/9 -> Conversion Transmission State/1
  Conversion Accuracy/1 -> Bus Creator/8  "Accuracy"
  Demux/8 -> Conversion Accuracy/1
  Conversion Elevation/1 -> Bus Creator/7  "Elevation"
  Demux/7 -> Conversion Elevation/1
  Conversion Longitudinal/1 -> Bus Creator/6  "Longitudinal"
  Demux/6 -> Conversion Longitudinal/1
  Conversion Lateral/1 -> Bus Creator/5  "Lateral"
  Demux/5 -> Conversion Lateral/1
  Conversion SecMark/1 -> Bus Creator/4  "SecMark"
  Demux/4 -> Conversion SecMark/1
  Conversion TempId/1 -> Bus Creator/3  "TempId"
  Demux/3 -> Conversion TempId/1
  Demux/2 -> Conversion MsgCount/1
  Conversion MsgCount/1 -> Bus Creator/2  "MsgCount"
  Bus Creator/1 -> Msg/1
  Conversion MsgId/1 -> Bus Creator/1  "MsgId"
  Demux/1 -> Conversion MsgId/1
  Data/1 -> Demux/1
  Always Enabled/1 -> f()/1

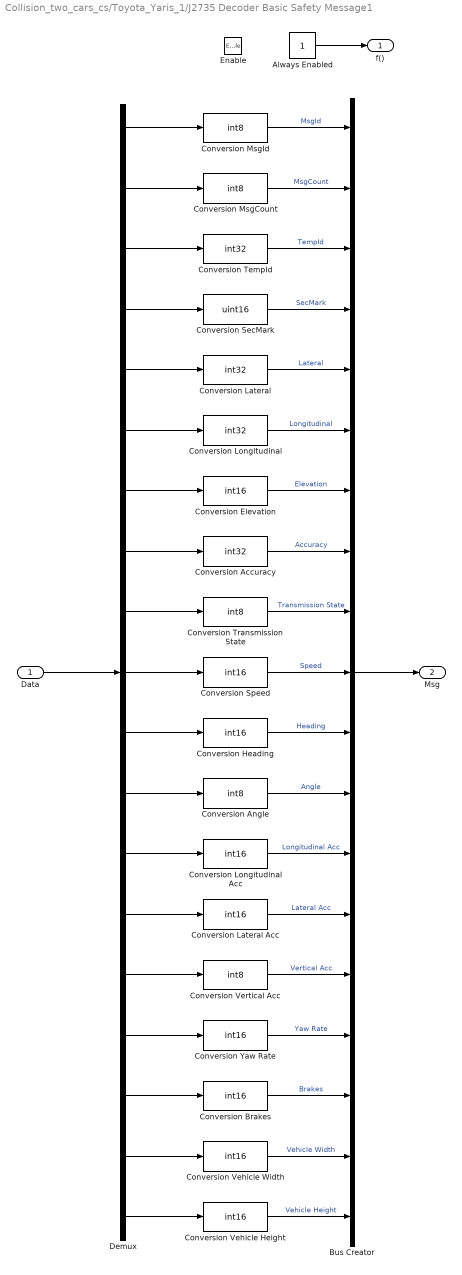
== system Collision_two_cars_cs/Toyota_Yaris_1/J2735 Decoder Basic Safety Message1 ==
  Data : Inport
  Enable : EnablePort  PropagateVarSize=During execution
  Always Enabled : Constant
  Bus Creator : BusCreator  Inputs=19
  Conversion Accuracy : DataTypeConversion  OutDataTypeStr=int32
  Conversion Angle : DataTypeConversion  OutDataTypeStr=int8
  Conversion Brakes : DataTypeConversion  OutDataTypeStr=int16
  Conversion Elevation : DataTypeConversion  OutDataTypeStr=int16
  Conversion Heading : DataTypeConversion  OutDataTypeStr=int16
  Conversion Lateral : DataTypeConversion  OutDataTypeStr=int32
  Conversion Lateral Acc : DataTypeConversion  OutDataTypeStr=int16
  Conversion Longitudinal : DataTypeConversion  OutDataTypeStr=int32
  Conversion Longitudinal Acc : DataTypeConversion  OutDataTypeStr=int16
  Conversion MsgCount : DataTypeConversion  OutDataTypeStr=int8
  Conversion MsgId : DataTypeConversion  OutDataTypeStr=int8
  Conversion SecMark : DataTypeConversion  OutDataTypeStr=uint16
  Conversion Speed : DataTypeConversion  OutDataTypeStr=int16
  Conversion TempId : DataTypeConversion  OutDataTypeStr=int32
  Conversion Transmission State : DataTypeConversion  OutDataTypeStr=int8
  Conversion Vehicle Height : DataTypeConversion  OutDataTypeStr=int16
  Conversion Vehicle Width : DataTypeConversion  OutDataTypeStr=int16
  Conversion Vertical Acc : DataTypeConversion  OutDataTypeStr=int8
  Conversion Yaw Rate : DataTypeConversion  OutDataTypeStr=int16
  Demux : Demux  Outputs=19
  f() : Outport  InitialOutput=[1]
  Msg : Outport  Port=2
  wires:
  Conversion Vehicle Height/1 -> Bus Creator/19  "Vehicle Height"
  Demux/19 -> Conversion Vehicle Height/1
  Conversion Vehicle Width/1 -> Bus Creator/18  "Vehicle Width"
  Conversion Brakes/1 -> Bus Creator/17  "Brakes"
  Demux/18 -> Conversion Vehicle Width/1
  Demux/17 -> Conversion Brakes/1
  Conversion Yaw Rate/1 -> Bus Creator/16  "Yaw Rate"
  Conversion Vertical Acc/1 -> Bus Creator/15  "Vertical Acc"
  Demux/16 -> Conversion Yaw Rate/1
  Demux/15 -> Conversion Vertical Acc/1
  Conversion Lateral Acc/1 -> Bus Creator/14  "Lateral Acc"
  Conversion Longitudinal Acc/1 -> Bus Creator/13  "Longitudinal Acc"
  Demux/14 -> Conversion Lateral Acc/1
  Demux/13 -> Conversion Longitudinal Acc/1
  Conversion Angle/1 -> Bus Creator/12  "Angle"
  Conversion Heading/1 -> Bus Creator/11  "Heading"
  Demux/12 -> Conversion Angle/1
  Demux/11 -> Conversion Heading/1
  Conversion Speed/1 -> Bus Creator/10  "Speed"
  Conversion Transmission State/1 -> Bus Creator/9  "Transmission State"
  Demux/10 -> Conversion Speed/1
  Demux/9 -> Conversion Transmission State/1
  Conversion Accuracy/1 -> Bus Creator/8  "Accuracy"
  Demux/8 -> Conversion Accuracy/1
  Conversion Elevation/1 -> Bus Creator/7  "Elevation"
  Demux/7 -> Conversion Elevation/1
  Conversion Longitudinal/1 -> Bus Creator/6  "Longitudinal"
  Demux/6 -> Conversion Longitudinal/1
  Conversion Lateral/1 -> Bus Creator/5  "Lateral"
  Demux/5 -> Conversion Lateral/1
  Conversion SecMark/1 -> Bus Creator/4  "SecMark"
  Demux/4 -> Conversion SecMark/1
  Conversion TempId/1 -> Bus Creator/3  "TempId"
  Demux/3 -> Conversion TempId/1
  Demux/2 -> Conversion MsgCount/1
  Conversion MsgCount/1 -> Bus Creator/2  "MsgCount"
  Bus Creator/1 -> Msg/1
  Conversion MsgId/1 -> Bus Creator/1  "MsgId"
  Demux/1 -> Conversion MsgId/1
  Data/1 -> Demux/1
  Always Enabled/1 -> f()/1

== system Collision_two_cars_cs/Toyota_Yaris_1/SELF_Demux ==
  SELF : Inport
  Demux1 : Demux  Outputs=3
  Demux2 : Demux  Outputs=3
  Demux3 : Demux  Outputs=[3 3 1 1]
  Demux4 : Demux  Outputs=3
  Gain : Gain  Gain=180/pi
  Gain1 : Gain  Gain=180/pi
  Selector : Selector  InputPortWidth=3  IndexOptions=Index vector (dialog)  Indices=[3]  OutputSizes=1
  compas converter : Subsystem
  xyz2GPS : PreScanUsefulBlocks/xyz2GPS  CoordinateCount=1  GPS_base=[48.534599 9.071365 0.000]
  x [m] : Outport
  y [m] : Outport  Port=2
  z [m] : Outport  Port=3
  rotx [deg] : Outport  Port=4
  roty [deg] : Outport  Port=5
  rotz [deg] : Outport  Port=6
  GPS lat [deg] : Outport  Port=7
  GPS long [deg] : Outport  Port=8
  GPS alt [m] : Outport  Port=9
  velocity [m/s] : Outport  Port=10
  heading [deg] : Outport  Port=11
  yaw rate [deg/s] : Outport  Port=12
  wires:
  Demux3/4 -> Gain1/1
  Gain1/1 -> yaw rate [deg/s]/1
  Demux3/3 -> velocity [m/s]/1
  compas converter/1(heading [deg]) -> heading [deg]/1
  xyz2GPS/1 -> Demux4/1
  Demux4/3 -> GPS alt [m]/1
  Demux4/2 -> GPS long [deg]/1
  Demux4/1 -> GPS lat [deg]/1
  Demux3/2 -> Gain/1, Selector/1
  Demux3/1 -> xyz2GPS/1, Demux1/1
  SELF/1 -> Demux3/1
  Demux2/3 -> rotz [deg]/1
  Demux2/2 -> roty [deg]/1
  Demux2/1 -> rotx [deg]/1
  Demux1/3 -> z [m]/1
  Demux1/2 -> y [m]/1
  Demux1/1 -> x [m]/1
  Gain/1 -> Demux2/1
  Selector/1 -> compas converter/1(rotz [rad])

== system Collision_two_cars_cs/Toyota_Yaris_1/Trajectories ==
  Traj2State1 : Subsystem  Tag=Traj2State  mask(PreScan Demux Block:){}
      settings: DeleteFcn=PreScanBlockDeleteFcn;
  Trajectory_3 : Subsystem  Tag=Trajectory  mask(PreScan Source Block: Trajectory){FileName='Trajectory_3_Synced.mat', TimeStep=1/20}
      mask prompts: TimeStep "Time Step [s]"
      mask help:
      | The Trajectory block contains the trajectories defined in the PreScan Experiment Editor. The output of the trajectory block is the (vehicle) State.
      |
      | For more information, please click Help.
      mask init: same as Collision_two_cars_cs/Audi_A8_1/Trajectories/Trajectory_1
      settings: DeleteFcn=PreScanBlockDeleteFcn;
      mask Help: eval('openHelp(312)')
      mask Display: fprintf(FileName)
  Trajectory_3_Offset : Constant  Tag=TrajectoryOffset  Value="[0  0  0  0  0  0]"
  State : Outport  Tag=TrajOutport
  wires:
  Trajectory_3/1(trajectory) -> Traj2State1/1(Traj Org)
  Trajectory_3_Offset/1 -> Traj2State1/2(Offset)
  Traj2State1/1(state) -> State/1

== system Collision_two_cars_cs/Audi_A8_1/AIR_1_Demux/Activate_Switch ==
  BeamID : Inport
  Heading : Inport  Port=2
  Constant : Constant  Value=0
  Product1 : Product  RndMeth=Zero
  Relational Operator : RelationalOperator  Operator=~=  OutDataTypeStr=boolean
  On/Off : Outport
  wires:
  Constant/1 -> Relational Operator/1
  Relational Operator/1 -> Product1/1
  BeamID/1 -> Relational Operator/2
  Product1/1 -> On/Off/1
  Heading/1 -> Product1/2

== system Collision_two_cars_cs/Audi_A8_1/AIR_1_Demux/Signal2ArrayOfSignals1 ==
  note: Set mask parameter VECTORLENGTH
      |  to MAXMESSAGES
  note: Initial state of Previous vector block
      | set to zeros(VECTORLENGTH,1)
  LoopIndex : Inport
  Element : Inport  Port=2
  Assignment : Assignment  IndexOptions=Index vector (port)  Indices=1  OutputSizes=1
  Previous vector : Memory  X0=zeros(VECTORLENGTH,1)  InheritSampleTime=on
  ArrayofElements : Outport
  wires:
  Element/1 -> Assignment/2
  LoopIndex/1 -> Assignment/3
  Previous vector/1 -> Assignment/1
  Assignment/1 -> ArrayofElements/1, Previous vector/1

== system Collision_two_cars_cs/Audi_A8_1/AIR_1_Demux/Signal2ArrayOfSignals2 ==
  note: Set mask parameter VECTORLENGTH
      |  to MAXMESSAGES
  note: Initial state of Previous vector block
      | set to zeros(VECTORLENGTH,1)
  LoopIndex : Inport
  Element : Inport  Port=2
  Assignment : Assignment  IndexOptions=Index vector (port)  Indices=1  OutputSizes=1
  Previous vector : Memory  X0=zeros(VECTORLENGTH,1)  InheritSampleTime=on
  ArrayofElements : Outport
  wires:
  Element/1 -> Assignment/2
  LoopIndex/1 -> Assignment/3
  Previous vector/1 -> Assignment/1
  Assignment/1 -> ArrayofElements/1, Previous vector/1

== system Collision_two_cars_cs/Audi_A8_1/AIR_1_Demux/Signal2ArrayOfSignals3 ==
  note: Set mask parameter VECTORLENGTH
      |  to MAXMESSAGES
  note: Initial state of Previous vector block
      | set to zeros(VECTORLENGTH,1)
  LoopIndex : Inport
  Element : Inport  Port=2
  Assignment : Assignment  IndexOptions=Index vector (port)  Indices=1  OutputSizes=1
  Previous vector : Memory  X0=zeros(VECTORLENGTH,1)  InheritSampleTime=on
  ArrayofElements : Outport
  wires:
  Element/1 -> Assignment/2
  LoopIndex/1 -> Assignment/3
  Previous vector/1 -> Assignment/1
  Assignment/1 -> ArrayofElements/1, Previous vector/1

== system Collision_two_cars_cs/Audi_A8_1/AIR_1_Demux/Signal2ArrayOfSignals4 ==
  note: Set mask parameter VECTORLENGTH
      |  to MAXMESSAGES
  note: Initial state of Previous vector block
      | set to zeros(VECTORLENGTH,1)
  LoopIndex : Inport
  Element : Inport  Port=2
  Assignment : Assignment  IndexOptions=Index vector (port)  Indices=1  OutputSizes=1
  Previous vector : Memory  X0=zeros(VECTORLENGTH,1)  InheritSampleTime=on
  ArrayofElements : Outport
  wires:
  Element/1 -> Assignment/2
  LoopIndex/1 -> Assignment/3
  Previous vector/1 -> Assignment/1
  Assignment/1 -> ArrayofElements/1, Previous vector/1
